simulink model "Aufgabe_10_2_7_Silos_und_Abfuellstation"  (R2023a)
settings: Solver=ode3  StartTime=0.0  StopTime=40  FixedStep=0.01  RelTol=1e-3  EnableMultiTasking=on
libraries: simulink x6
settings Model: Creator=SimTP16  LastModifiedBy=ASUS
settings SolverCC: AlgebraicLoopSolver=TrustRegion
settings DataIOCC: LimitDataPoints=on  SaveFormat=Array  ReturnWorkspaceOutputs=off
settings OptimizationCC: LifeSpan=inf
settings DebuggingCC: UnderspecifiedInitializationDetection=Classic  MergeDetectMultiDrivingBlocksExec=none  SolverPrmCheckMsg=warning  UnconnectedInputMsg=warning  UnconnectedOutputMsg=warning  UnconnectedLineMsg=warning  StateNameClashWarn=warning  SFUnexpectedBacktrackingDiag=warning  SFNoUnconditionalDefaultTransitionDiag=warning  SFExecutionAtInitializationDiag=none  ArithmeticOperatorsInVariantConditions=warning
settings HardwareCC: ProdBitPerPointer=32  ProdBitPerSizeT=32  ProdBitPerPtrDiffT=32  ProdLargestAtomicFloat=None  ProdIntDivRoundTo=Undefined  ProdEndianess=Unspecified  ProdWordSize=32  ProdHWDeviceType=32-bit Generic
settings ModelReferenceCC: PropagateSignalLabelsOutOfModel=off
settings SFSimCC: SimUseLocalCustomCode=off  CustomCodeUndefinedFunction=UseInterfaceOnly
settings RTWCC: RTWUseLocalCustomCode=off
settings CodeAppCC: StateflowObjectComments=on
settings GRTTargetCC: TargetLangStandard=C89/C90 (ANSI)
settings ConfigComp: CovMetricSettings=dw  CovSaveCumulativeToWorkspaceVar=on  CovSaveSingleToWorkspaceVar=on  CovExternalEMLEnable=off

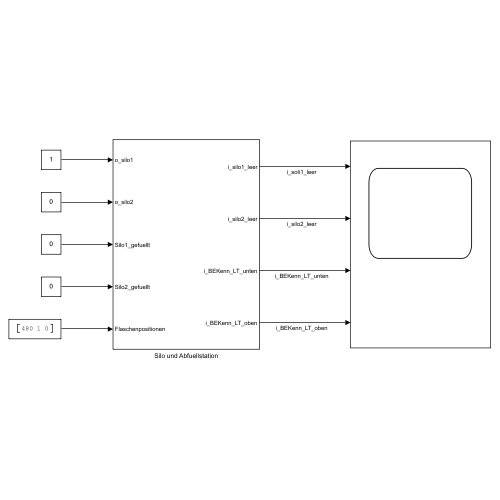
[thumbnail: Simulink's stored preview of the top-level diagram]
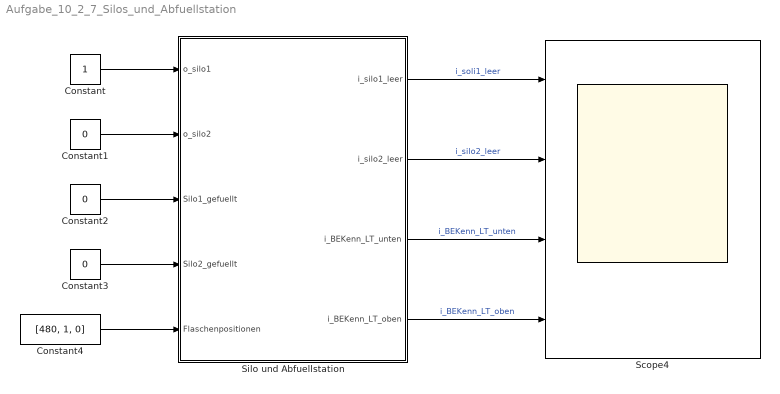
== system Aufgabe_10_2_7_Silos_und_Abfuellstation ==
  Constant : Constant
  Constant1 : Constant  Value=0
  Constant2 : Constant  Value=0
  Constant3 : Constant  Value=0
  Constant4 : Constant  Value=[480, 1, 0]
  Scope4 : Scope  NumInputPorts=4
  Silo und Abfuellstation : Subsystem
  wires:
  Silo und Abfuellstation/4(i_BEKenn_LT_oben) -> Scope4/4  "i_BEKenn_LT_oben"
  Silo und Abfuellstation/3(i_BEKenn_LT_unten) -> Scope4/3  "i_BEKenn_LT_unten"
  Silo und Abfuellstation/2(i_silo2_leer) -> Scope4/2  "i_silo2_leer"
  Silo und Abfuellstation/1(i_silo1_leer) -> Scope4/1  "i_soli1_leer"
  Constant1/1 -> Silo und Abfuellstation/2(o_silo2)
  Constant/1 -> Silo und Abfuellstation/1(o_silo1)
  Constant2/1 -> Silo und Abfuellstation/3(Silo1_gefuellt)
  Constant3/1 -> Silo und Abfuellstation/4(Silo2_gefuellt)
  Constant4/1 -> Silo und Abfuellstation/5(Flaschenpositionen)

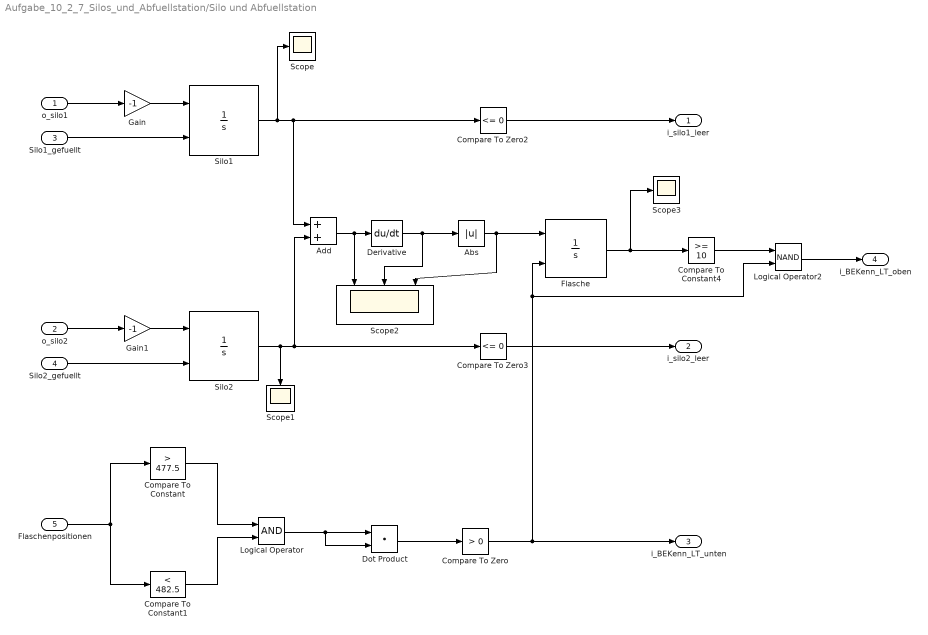
== system Aufgabe_10_2_7_Silos_und_Abfuellstation/Silo und Abfuellstation ==
  o_silo1 : Inport
  o_silo2 : Inport  Port=2
  Silo1_gefuellt : Inport  Port=3
  Silo2_gefuellt : Inport  Port=4
  Flaschenpositionen : Inport  Port=5
  Abs : Abs  SaturateOnIntegerOverflow=off
  Add : Sum
  Compare To Constant : simulink/Logic and Bit Operations/Compare To Constant  relop=>  const=477.5  OutDataTypeStr=boolean
  Compare To Constant1 : simulink/Logic and Bit Operations/Compare To Constant  relop=<  const=482.5  OutDataTypeStr=boolean
  Compare To Constant4 : simulink/Logic and Bit Operations/Compare To Constant  relop=>=  const=10  OutDataTypeStr=boolean
  Compare To Zero : simulink/Logic and Bit Operations/Compare To Zero  relop=>  OutDataTypeStr=boolean
  Compare To Zero2 : simulink/Logic and Bit Operations/Compare To Zero  relop=<=  OutDataTypeStr=boolean
  Compare To Zero3 : simulink/Logic and Bit Operations/Compare To Zero  relop=<=  OutDataTypeStr=boolean
  Derivative : Derivative
  Dot Product : DotProduct  OutDataTypeStr=Inherit: Inherit via internal rule
  Flasche : Integrator  ExternalReset=falling  LimitOutput=on  UpperSaturationLimit=10  LowerSaturationLimit=0
  Gain : Gain  Gain=-1
  Gain1 : Gain  Gain=-1
  Logical Operator : Logic  AllPortsSameDT=off  OutDataTypeStr=boolean
  Logical Operator2 : Logic  Operator=NAND  AllPortsSameDT=off  OutDataTypeStr=boolean
  Scope : Scope
  Scope1 : Scope
  Scope2 : Scope  NumInputPorts=3
  Scope3 : Scope
  Silo1 : Integrator  ExternalReset=rising  InitialCondition=10  LimitOutput=on  UpperSaturationLimit=10  LowerSaturationLimit=0
  Silo2 : Integrator  ExternalReset=rising  InitialCondition=10  LimitOutput=on  UpperSaturationLimit=10  LowerSaturationLimit=0
  i_silo1_leer : Outport
  i_silo2_leer : Outport  Port=2
  i_BEKenn_LT_unten : Outport  Port=3
  i_BEKenn_LT_oben : Outport  Port=4
  wires:
  o_silo2/1 -> Gain1/1
  Compare To Zero2/1 -> i_silo1_leer/1
  o_silo1/1 -> Gain/1
  Compare To Zero3/1 -> i_silo2_leer/1
  Logical Operator2/1 -> i_BEKenn_LT_oben/1
  Gain1/1 -> Silo2/1
  Silo2/1 -> Scope1/1, Add/2, Compare To Zero3/1
  Flasche/1 -> Scope3/1, Compare To Constant4/1
  Add/1 -> Scope2/1, Derivative/1
  Silo1/1 -> Scope/1, Add/1, Compare To Zero2/1
  Gain/1 -> Silo1/1
  Dot Product/1 -> Compare To Zero/1
  Compare To Zero/1 -> Logical Operator2/2, Flasche/2, i_BEKenn_LT_unten/1
  Flaschenpositionen/1 -> Compare To Constant1/1, Compare To Constant/1
  Compare To Constant1/1 -> Logical Operator/2
  Logical Operator/1 -> Dot Product/2, Dot Product/1
  Compare To Constant/1 -> Logical Operator/1
  Compare To Constant4/1 -> Logical Operator2/1
  Silo1_gefuellt/1 -> Silo1/2
  Silo2_gefuellt/1 -> Silo2/2
  Derivative/1 -> Scope2/2, Abs/1
  Abs/1 -> Scope2/3, Flasche/1
